simulink model "simulazione_sistema_osservatore_errore_uscita"  (R2019b)
settings: Solver=VariableStepAuto  StartTime=0.0  StopTime=10.0  RelTol=1e-3
values from neighbouring files (symbols this model uses):
  B = [0;0;1/m1;0]    [ValoriCaso1.m]    (also in ValoriCaso2.m; ValoriCaso3.m; ValoriCaso4.m; ValoriCaso5.m)
  c = 0    [ValoriCaso1.m]    (also in ValoriCaso2.m = 2; ValoriCaso3.m = 5; ValoriCaso4.m; ValoriCaso5.m = 2)
  k = 2    [ValoriCaso1.m]    (also in ValoriCaso2.m = 4; ValoriCaso3.m = 4; ValoriCaso4.m; ValoriCaso5.m = 4)
  m1 = 1    [ValoriCaso1.m]    (also in ValoriCaso2.m = 2; ValoriCaso3.m = 2; ValoriCaso4.m; ValoriCaso5.m = 2)
  m2 = 1    [ValoriCaso1.m]    (also in ValoriCaso2.m = 2; ValoriCaso3.m = 2; ValoriCaso4.m; ValoriCaso5.m = 2)
  mat_S = A-(V*C)    [CreazioneOsservatore.m]
  V = -(Fd')    [CreazioneOsservatore.m]
  x0 = [0;10;0;0]    [ValoriCaso1.m]    (also in ValoriCaso2.m; ValoriCaso3.m; ValoriCaso4.m; ValoriCaso5.m)
settings Model: Creator=sugam  LastModifiedBy=sugam

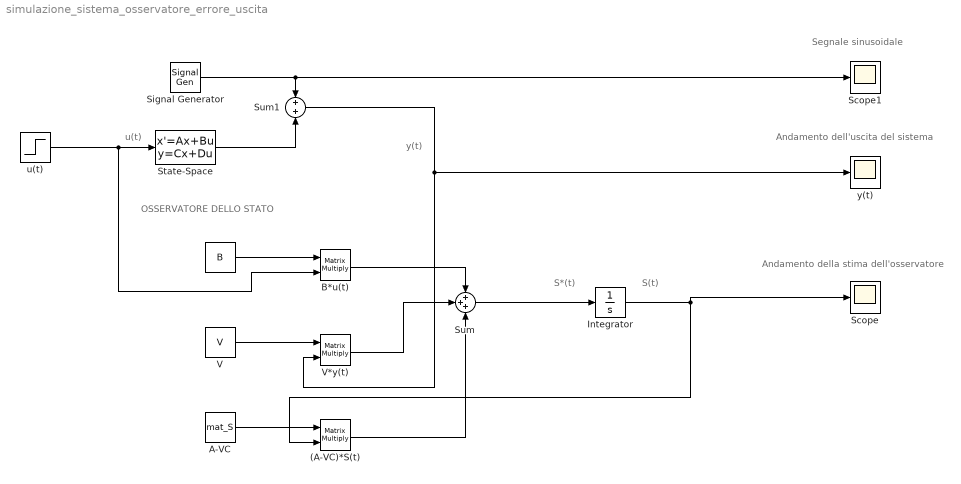
== system simulazione_sistema_osservatore_errore_uscita ==
  note: Segnale sinusoidale
  note: OSSERVATORE DELLO STATO
  note: y(t)
  note: S(t)
  note: S*(t)
  note: u(t)
  note: Andamento della stima dell'osservatore
  note: Andamento dell'uscita del sistema
  " " : Constant  Value=B  SampleTime=0
  (A-VC)*S(t) : Product  Multiplication=Matrix(*)
  A-VC : Constant  Value=mat_S  VectorParams1D=off  SampleTime=0
  B*u(t) : Product  Multiplication=Matrix(*)
  Integrator : Integrator
  Scope : Scope
  Scope1 : Scope
  Signal Generator : SignalGenerator  Frequency=3  VectorParams1D=off
  State-Space : StateSpace  A=[0 0 1 0;0 0 0 1;-k/m1 k/m1 -c/m1 c/m1;k/m2 -k/m2 c/m2 -c/m2]  B=[0;0;1/m1;0]  C=[1 0 0 0]  D=0  InitialCondition=x0
  Sum : Sum  Inputs=+++
  Sum1 : Sum
  V : Constant  Value=V  VectorParams1D=off  SampleTime=0
  V*y(t) : Product  Multiplication=Matrix(*)
  u(t) : Step  Time=0  After=5  SampleTime=0  VectorParams1D=off
  y(t) : Scope
  wires:
  " "/1 -> B*u(t)/1
  A-VC/1 -> (A-VC)*S(t)/1
  u(t)/1 -> State-Space/1, B*u(t)/2
  Sum/1 -> Integrator/1
  V*y(t)/1 -> Sum/2
  B*u(t)/1 -> Sum/1
  (A-VC)*S(t)/1 -> Sum/3
  V/1 -> V*y(t)/1
  Integrator/1 -> Scope/1, (A-VC)*S(t)/2
  Signal Generator/1 -> Scope1/1, Sum1/1
  State-Space/1 -> Sum1/2
  Sum1/1 -> V*y(t)/2, y(t)/1
